simulink model "vector_quantizer_example"  (Simulink 6.0)
settings: Solver=FixedStepDiscrete  SolverMode=SingleTasking  StartTime=0.0  StopTime=0.49  RelTol=1e-3
PreLoadFcn:
  | load mtlb;
undefined symbols (not defined in the file or in its folder): Mag, magnitude, mtlb
libraries: simulink x6, dspquant2 x6, dspsnks4 x5, dspsrcs4 x4, dsparch4 x4, dsplp x4, dspmathops x3, dspmtrx3 x3, dspstat3 x2, dspindex x2, dspsigops x2, dspxfrm3 x1
settings Model: RequirementInfo=9  CovMetricSettings=d  Creator=dshpak  LastModifiedBy=cclarke  ExtModeTrigMode=oneshot  ExtModeArmWhenConnect=off  ExtModeAutoUpdateStatusClock=off  SaveTime=off  SaveOutput=off  SaveFormat=Structure  LimitDataPoints=off  IntegerOverflowMsg=none  BlockReductionOpt=off  ZeroCrossControl=UseLocalSettings  ProdHWDeviceType=Microprocessor  TargetHWChar=2  TargetHWWordLengths=8,16,32,32  RTWMathFcnLibMatFile=iso_c_tmw.mat  RTWOptions="-aEnforceIntegerDowncast=1 -aFoldNonRolledExpr=1 -aInlineInvariantSignals=0 -aInlineParameters=0 -aLocalBlockOutputs=1 -aRollThreshold=5 -aGenerateReport=0 -aGenCodeOnly=0 -aRTWVerbose=1 -aForceParamTrailComments=0 -aGenerateComments=1 -aIgnoreCustomStorageClasses=1 -aIncHierarchyInIds=0 -aMaxRTWIdLen=31 -aShowEliminatedStatements=1 -aPrefixModelToSubsysFcnNames=1 -aIncDataTypeInIds=0 -aInlinedPrmAccess=\"Literals\" -aTargetFcnLib=\"iso_c_tmw.mat\" -aGenerateFullHeader=1 -aIsPILTarget=0 -aExtMode=0 -aExtModeStaticAlloc=0 -aExtModeTesting=0 -aExtModeStaticAllocSize=1000000 -aExtModeTransport=0 -aLogVarNameModifier=\"rt_\" -aRTWCAPISignals=0 -aRTWCAPIParams=0"
settings DataIOCC: LimitDataPoints=off  SaveFormat=Structure  SaveOutput=off  SaveTime=off  SignalLoggingName=sigsOut
settings OptimizationCC: BlockReduction=off  BooleanDataType=off  InlineInvariantSignals=off  MultiInstanced=off
settings FormatCC: IgnoreBidirectionalLines=off
settings DebuggingCC: IntegerOverflowMsg=none
settings HardwareCC: ProdHWDeviceType=Microprocessor  ShiftRightIntArith=on  TargetHWCharacteristics=InheritFromRTWHook
settings CodeAppCC: FileBanners=off
settings GRTTargetCC: TargetFcnLib=iso_c_tmw.mat  IsERTTarget=off

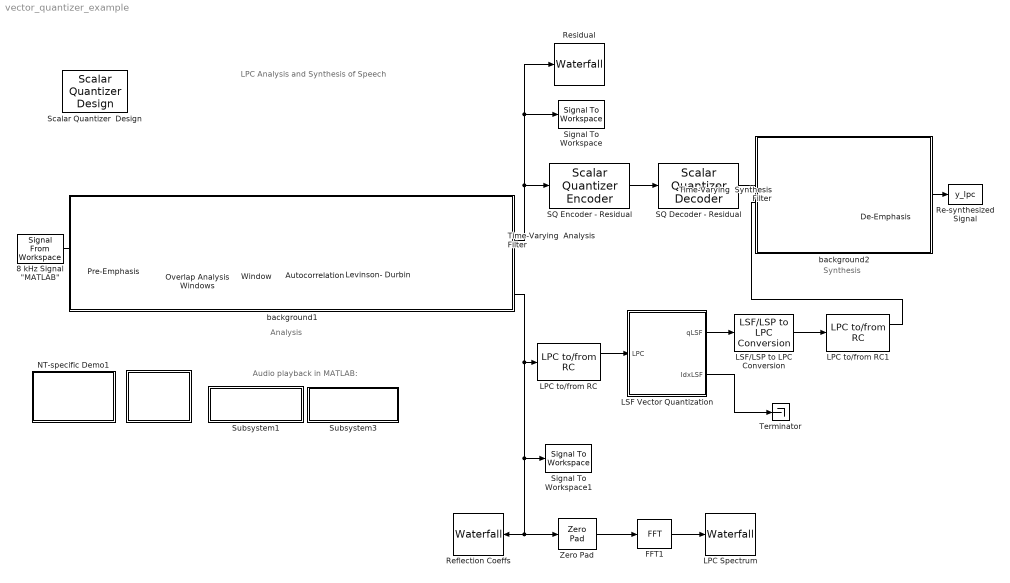
== system vector_quantizer_example ==
  note: LPC Analysis and Synthesis of Speech
  note: Analysis
  note: Synthesis
  note: Audio playback in MATLAB:
  " " : Subsystem
      mask Type: Frame-Based Simulation Info
      mask Display: disp('Info')
  "8 kHz Signal \"MATLAB\"" : dspsrcs4/Signal From Workspace  X=mtlb*0.32  Ts=1/8000  nsamps=80  OutputAfterFinalValue=Setting to zero
  Autocorrelation : dspstat3/Autocorrelation  AllPositiveLags=off  maxlag=12  bias=Biased  domain=Time  roundingMode=Floor  overflowMode=off
  De-Emphasis : dsparch4/Digital Filter  TypePopup=IIR (all poles)  IIRFiltStruct=Direct form II transposed  AllPoleFiltStruct=Direct form  FIRFiltStruct=Direct form  CoeffSource=Specify via dialog  NumCoeffs=[1 -.95]  DenCoeffs=[1 -.95]  BiQuadCoeffs=[1 0.3 0.4 1 0.1 0.2]  LatticeCoeffs=[0.2 0.4]  denIgnore=on  FiltPerSampPopup=One filter per frame  IC=0  ICnum=0  ICden=0  roundingMode=Floor  overflowMode=off
  FFT1 : dspxfrm3/FFT  CompMethod=Table lookup  TableOpt=Speed  BitRevOrder=off  SkipNorm=off  roundingMode=Floor  overflowMode=off
  LPC Spectrum : dspsnks4/Waterfall  TraceProperties=off  NumTraces=10  CMapStr=autumn  TNewest=0.35  TOldest=0.1  HistoryLength=100  HistoryFull=Overwrite  UpdateInterval=1  ExportMode=All visible  MLExportName=ExportData  AutoExport=off  DisplayProperties=off  MouseMode=Orbit  AxisGrid=off  Snapshot=off  Suspend=off  SyncSnapshots=off  OpenScopeAtSimStart=off  FigPos=[452 44 407 353]  CameraView=[89945.9047576273 49093.2447020758 -7462.52930692949 -16.6995606364064 71 5.5 2.5389885178677 -5.30668596526891 0.808418434368868 0.0592442608385446 5.583225828012 14.2 1]  InportDimsHint=[129 1]  AxisProperties=off  AxisColor=[1 1 1]*.9  XLabel=Frequency  YLabel=Mag^2  ZLabel=History  TriggerProperties=off  TrigStartMode=Immediately  TrigStartT=10  TrigStartN=1000  TrigStartFcn=trigPower  TrigStopMode=Never  TrigStopT=0.1  TrigStopN=10  TrigStopFcn=trigend  TrigRearmMode=User-defined  TrigRearmT=0  TrigRearmN=100  TrigRearmFcn=trigrearm  XformProperties=off  XformMode=FFT->Mag dB Fs/2  XformFcn=fliplr  XformExpr=20*log10(abs(u(129:2:end)))
      settings: YMin=-44.6156897764664  YMax=11.2165685036536
  LPC to/from RC : dsplp/LPC to//from RC  conversion=RC to LPC  perr=on  stability=off  error=Replace it with 1
  LPC to/from RC1 : dsplp/LPC to//from RC  conversion=RC to LPC  perr=on  stability=off  error=Replace it with 1
  LSF Vector Quantization : Subsystem
  LSF/LSP to LPC Conversion : dsplp/LSF//LSP to LPC Conversion  input=LSP in range (-1 1)
  Levinson- Durbin : dspsolvers/Levinson-Durbin  coeffOutFcn=K  outP=off  zeroInpHandling=on
  NT-specific Demo1 : Subsystem
      settings: OpenFcn=dsplpc_win32
      mask Type: NT-only Demo
      mask Display: disp('PC/Windows\nLPC Demo')
  Overlap Analysis Windows : dspbuff3/Buffer  N=160  V=80  ic=0
  Pre-Emphasis : dsparch4/Digital Filter  TypePopup=FIR (all zeros)  IIRFiltStruct=Direct form II transposed  AllPoleFiltStruct=Direct form  FIRFiltStruct=Direct form  CoeffSource=Specify via dialog  NumCoeffs=[1 -.95]  DenCoeffs=[1 0.1]  BiQuadCoeffs=[1 0.3 0.4 1 0.1 0.2]  LatticeCoeffs=[0.2 0.4]  denIgnore=on  FiltPerSampPopup=One filter per frame  IC=0  ICnum=0  ICden=0  roundingMode=Floor  overflowMode=off
  Re-synthesized Signal : ToWorkspace  VariableName=y_lpc  SampleTime=-1  SaveFormat=Array
  Reflection Coeffs : dspsnks4/Waterfall  Orientation=left  TraceProperties=off  NumTraces=10  CMapStr=autumn  TNewest=0.7  TOldest=0.1  HistoryLength=50  HistoryFull=Overwrite  UpdateInterval=1  ExportMode=All visible  MLExportName=ExportData2  AutoExport=off  DisplayProperties=off  MouseMode=Orbit  AxisGrid=on  Snapshot=off  Suspend=off  SyncSnapshots=off  OpenScopeAtSimStart=off  FigPos=[35 41 410 358]  CameraView=[73343.0440471642 150383.489958622 -231607.055769344 -0.0735265549347769 7.5 5.5 0.547487828138618 -2.62241953831449 4.03911084299836 0.00240035045613671 1 7.88928028685195 5.25952019123463]  InportDimsHint=[12 1]  AxisProperties=off  AxisColor=[1 1 1]*.9  XLabel=Coefficient  YLabel=RC Amplitude  ZLabel=History  TriggerProperties=off  TrigStartMode=Immediately  TrigStartT=10  TrigStartN=1000  TrigStartFcn=trigPower  TrigStopMode=Never  TrigStopT=0.1  TrigStopN=10  TrigStopFcn=trigend  TrigRearmMode=User-defined  TrigRearmT=0  TrigRearmN=100  TrigRearmFcn=trigrearm  XformProperties=off  XformMode=None  XformFcn=fliplr  XformExpr=20*log10(abs(u(129:2:end)))
      settings: YMin=-1.02418361455266  YMax=0.877130504683106
  Residual : dspsnks4/Waterfall  TraceProperties=off  NumTraces=10  CMapStr=autumn  TNewest=0.7  TOldest=0.1  HistoryLength=50  HistoryFull=Overwrite  UpdateInterval=1  ExportMode=All visible  MLExportName=ExportData2  AutoExport=off  DisplayProperties=off  MouseMode=Orbit  AxisGrid=on  Snapshot=off  Suspend=off  SyncSnapshots=off  OpenScopeAtSimStart=off  FigPos=[524 276 410 358]  CameraView=[62164.2347969079 1792549.89917746 -405278.370332737 -0.097024155318337 44.5 5.5 0.575539043328793 -33.5051317778483 7.57548038023531 0.00104183380472551 1 92.0645761641202 10.3443344004629]  InportDimsHint=[80 1]  AxisProperties=off  AxisColor=[1 1 1]*.9  XLabel=Coefficient  YLabel=Amplitude  ZLabel=History  TriggerProperties=off  TrigStartMode=Immediately  TrigStartT=10  TrigStartN=1000  TrigStartFcn=trigPower  TrigStopMode=Never  TrigStopT=0.1  TrigStopN=10  TrigStopFcn=trigend  TrigRearmMode=User-defined  TrigRearmT=0  TrigRearmN=100  TrigRearmFcn=trigrearm  XformProperties=off  XformMode=None  XformFcn=fliplr  XformExpr=20*log10(abs(u(129:2:end)))
      settings: YMin=-0.580380532484202  YMax=0.386332221847528
  SQ Decoder - Residual : dspquant2/Scalar Quantizer Decoder  Tag=SQDESIGN_GUI_REALIZE_MODEL  CBsource=Specify via dialog  codebook="[-0.52762    -0.50434    -0.48686    -0.48023    -0.47847      -0.471    -0.46439    -0.45511     -0.4483    -0.44149    -0.41351    -0.40777    -0.38649    -0.38257    -0.34459    -0.33656      -0.332    -0.31506     -0.3058    -0.29467    -0.28964    -0.27695    -0.26405    -0.25569    -0.24792    -0.24257    -0.23586    -0.22862     -0.2106    -0.20577    -0.20412    -0.18901    -0.18326    -0.17976    -0.17701    -0.17353    -0.16764    -0.16375    -0.15999    -0.15604    -0.15179    -0.14868    -0.14379    -0.13796    -0.13635    -0.13256    -0.13017    -0.12998    -0.12647    -0.12418    -0.11813     -0.1136    -0.11155    -0.11052    -0.10963    -0.10743    -0.10473    -0.10243     -0.1011   -0.099393   -0.096895   -0.094117   -0.089935   -0.085798   -0.081628   -0.076302   -0.068999   -0.061675   -0.053416   -0.045539   -0.039235   -0.031285   -0.023645   -0.016735   -0.011309  -0.0064137  -0.0017528   0.0031653   0.0083379    0.013857    0.020398      0.0273    0.035732    0.044282    0.051892    0.058205    0.064287    0.068767    0.072477     0.07818    0.082855    0.086893    0.093341     0.10139     0.10818     0.11338     0.12005      0.1266      0.1299     0.13376     0.13746     0.14153     0.14549     0.14866     0.14958     0.15164     0.15552     0.15703     0.15896     0.16211      0.1658     0.16848     0.17145     0.17815      0.1849      0.1891     0.19733     0.20475     0.20935     0.21575     0.22642     0.23266     0.23916     0.24329     0.25005      0.2589     0.27394     0.35121]"  invalidin=Clip  cwdtype=double  outputMode=User-defined  outputWordLength=16  outputFracLength=15
      settings: allowOverrides=off
  SQ Encoder - Residual : dspquant2/Scalar Quantizer Encoder  Tag=SQDESIGN_GUI_REALIZE_MODEL  paramSrc=Specify via dialog  partType=Bounded  BBoundary="[-inf -0.51598     -0.4956    -0.48355    -0.47935    -0.47473    -0.46769    -0.45975     -0.4517     -0.4449     -0.4275    -0.41064    -0.39713    -0.38453    -0.36358    -0.34057    -0.33428    -0.32353    -0.31043    -0.30024    -0.29216    -0.28329     -0.2705    -0.25987     -0.2518    -0.24524    -0.23922    -0.23224    -0.21961    -0.20819    -0.20495    -0.19656    -0.18613    -0.18151    -0.17839    -0.17527    -0.17058    -0.16569    -0.16187    -0.15802    -0.15392    -0.15024    -0.14624    -0.14088    -0.13716    -0.13446    -0.13136    -0.13007    -0.12823    -0.12533    -0.12115    -0.11587    -0.11258    -0.11103    -0.11007    -0.10853    -0.10608    -0.10358    -0.10176    -0.10024   -0.098144   -0.095506   -0.092026   -0.087867   -0.083713   -0.078965   -0.072651   -0.065337   -0.057545   -0.049477   -0.042387    -0.03526   -0.027465    -0.02019   -0.014022  -0.0088614  -0.0040832  0.00070626   0.0057516    0.011097    0.017127    0.023849    0.031516    0.040007    0.048087    0.055049    0.061246    0.066527    0.070622    0.075328    0.080518    0.084874    0.090117    0.097368     0.10479     0.11078     0.11671     0.12332     0.12825     0.13183     0.13561      0.1395     0.14351     0.14707     0.14912     0.15061     0.15358     0.15628       0.158     0.16054     0.16396     0.16714     0.16996      0.1748     0.18152       0.187     0.19321     0.20104     0.20705     0.21255     0.22109     0.22954     0.23591     0.24122     0.24667     0.25447     0.26642     0.31258  +inf]"  UBoundary="[ -0.51598     -0.4956    -0.48355    -0.47935    -0.47473    -0.46769    -0.45975     -0.4517     -0.4449     -0.4275    -0.41064    -0.39713    -0.38453    -0.36358    -0.34057    -0.33428    -0.32353    -0.31043    -0.30024    -0.29216    -0.28329     -0.2705    -0.25987     -0.2518    -0.24524    -0.23922    -0.23224    -0.21961    -0.20819    -0.20495    -0.19656    -0.18613    -0.18151    -0.17839    -0.17527    -0.17058    -0.16569    -0.16187    -0.15802    -0.15392    -0.15024    -0.14624    -0.14088    -0.13716    -0.13446    -0.13136    -0.13007    -0.12823    -0.12533    -0.12115    -0.11587    -0.11258    -0.11103    -0.11007    -0.10853    -0.10608    -0.10358    -0.10176    -0.10024   -0.098144   -0.095506   -0.092026   -0.087867   -0.083713   -0.078965   -0.072651   -0.065337   -0.057545   -0.049477   -0.042387    -0.03526   -0.027465    -0.02019   -0.014022  -0.0088614  -0.0040832  0.00070626   0.0057516    0.011097    0.017127    0.023849    0.031516    0.040007    0.048087    0.055049    0.061246    0.066527    0.070622    0.075328    0.080518    0.084874    0.090117    0.097368     0.10479     0.11078     0.11671     0.12332     0.12825     0.13183     0.13561      0.1395     0.14351     0.14707     0.14912     0.15061     0.15358     0.15628       0.158     0.16054     0.16396     0.16714     0.16996      0.1748     0.18152       0.187     0.19321     0.20104     0.20705     0.21255     0.22109     0.22954     0.23591     0.24122     0.24667     0.25447     0.26642     0.31258  ]"  SearchMethod=Binary  tieBreakRule=Choose the lower index  outQU=off  outQError=off  codebook="[-0.52762    -0.50434    -0.48686    -0.48023    -0.47847      -0.471    -0.46439    -0.45511     -0.4483    -0.44149    -0.41351    -0.40777    -0.38649    -0.38257    -0.34459    -0.33656      -0.332    -0.31506     -0.3058    -0.29467    -0.28964    -0.27695    -0.26405    -0.25569    -0.24792    -0.24257    -0.23586    -0.22862     -0.2106    -0.20577    -0.20412    -0.18901    -0.18326    -0.17976    -0.17701    -0.17353    -0.16764    -0.16375    -0.15999    -0.15604    -0.15179    -0.14868    -0.14379    -0.13796    -0.13635    -0.13256    -0.13017    -0.12998    -0.12647    -0.12418    -0.11813     -0.1136    -0.11155    -0.11052    -0.10963    -0.10743    -0.10473    -0.10243     -0.1011   -0.099393   -0.096895   -0.094117   -0.089935   -0.085798   -0.081628   -0.076302   -0.068999   -0.061675   -0.053416   -0.045539   -0.039235   -0.031285   -0.023645   -0.016735   -0.011309  -0.0064137  -0.0017528   0.0031653   0.0083379    0.013857    0.020398      0.0273    0.035732    0.044282    0.051892    0.058205    0.064287    0.068767    0.072477     0.07818    0.082855    0.086893    0.093341     0.10139     0.10818     0.11338     0.12005      0.1266      0.1299     0.13376     0.13746     0.14153     0.14549     0.14866     0.14958     0.15164     0.15552     0.15703     0.15896     0.16211      0.1658     0.16848     0.17145     0.17815      0.1849      0.1891     0.19733     0.20475     0.20935     0.21575     0.22642     0.23266     0.23916     0.24329     0.25005      0.2589     0.27394     0.35121]"  outStatus=off  invalidin=Clip  idtype=int32  roundingMode=Nearest  overflowMode=on
  Scalar Quantizer  Design : dspquant2/Scalar Quantizer  Design
  Signal To Workspace : dspsnks4/Signal To Workspace  VariableName=E  FrameMode=Concatenate frames (2-D array)
  Signal To Workspace1 : dspsnks4/Signal To Workspace  VariableName=K  FrameMode=Concatenate frames (2-D array)
  Subsystem1 : Subsystem
      settings: OpenFcn=if exist('mtlb','var'), sound(mtlb*0.32,8000); else errordlg('Data not found in workspace - reload demo model.','DSP Blockset Demo Error'); end
      mask Display: disp('Original\nSignal')
  Subsystem3 : Subsystem
      settings: OpenFcn=if exist('y_lpc','var'), sound(y_lpc,8000); else errordlg('You must run the simulation first.','DSP Blockset Demo Error'); end
      mask Display: disp('Processed\nSignal')
  Terminator : Terminator
  Time-Varying  Analysis Filter : dsparch4/Digital Filter  TypePopup=FIR (all zeros)  IIRFiltStruct=Direct form II transposed  AllPoleFiltStruct=Direct form  FIRFiltStruct=Lattice MA  CoeffSource=Input port(s)  NumCoeffs=[1 -.95]  DenCoeffs=[1 0.1]  BiQuadCoeffs=[1 0.3 0.4 1 0.1 0.2]  LatticeCoeffs=[0.2 0.4]  denIgnore=on  FiltPerSampPopup=One filter per frame  IC=0  ICnum=0  ICden=0  roundingMode=Floor  overflowMode=off
  Time-Varying  Synthesis Filter : dsparch4/Digital Filter  TypePopup=IIR (all poles)  IIRFiltStruct=Direct form II transposed  AllPoleFiltStruct=Lattice AR  FIRFiltStruct=Direct form  CoeffSource=Input port(s)  NumCoeffs=[1 -.95]  DenCoeffs=[1 0.1]  BiQuadCoeffs=[1 0.3 0.4 1 0.1 0.2]  LatticeCoeffs=[0.2 0.4]  denIgnore=on  FiltPerSampPopup=One filter per frame  IC=0  ICnum=0  ICden=0  roundingMode=Floor  overflowMode=off
  Window : dspsigops/Window Function  winmode=Apply window to input  wintype=Hamming  sampmode=Continuous  samptime=1  N=64  Rs=50  beta=10  winsamp=Symmetric  UserWindow=hamming  OptParams=off  UserParams={1.0}  dataType=double  wordLen=16  udDataType=sfix(16)  fracBitsMode=Best precision  numFracBits=15  roundingMode=Floor  overflowMode=off
  Zero Pad : dspsigops/Zero Pad  padSigAt=End  zpadAlong=Columns  padNumOutRowsSpecMethod=User-specified  numOutRows=256  padNumOutColsSpecMethod=User-specified  numOutCols=1  trunc_flag=None
  background1 : Subsystem
      mask Display: disp('')
  background2 : Subsystem
      mask Display: disp('')
  wires:
  "8 kHz Signal \"MATLAB\""/1 -> Pre-Emphasis/1
  Pre-Emphasis/1 -> Overlap Analysis Windows/1, Time-Varying  Analysis Filter/1
  Overlap Analysis Windows/1 -> Window/1
  Autocorrelation/1 -> Levinson- Durbin/1
  Window/1 -> Autocorrelation/1
  Time-Varying  Analysis Filter/1 -> Residual/1, Signal To Workspace/1, SQ Encoder - Residual/1
  Levinson- Durbin/1 -> Time-Varying  Analysis Filter/2, Reflection Coeffs/1, Zero Pad/1, Signal To Workspace1/1, LPC to/from RC/1
  Time-Varying  Synthesis Filter/1 -> De-Emphasis/1
  De-Emphasis/1 -> Re-synthesized Signal/1
  Zero Pad/1 -> FFT1/1
  FFT1/1 -> LPC Spectrum/1
  SQ Encoder - Residual/1 -> SQ Decoder - Residual/1
  SQ Decoder - Residual/1 -> Time-Varying  Synthesis Filter/1
  LSF Vector Quantization/2(IdxLSF) -> Terminator/1
  LPC to/from RC/1 -> LSF Vector Quantization/1(LPC)
  LSF Vector Quantization/1(qLSF) -> LSF/LSP to LPC Conversion/1
  LSF/LSP to LPC Conversion/1 -> LPC to/from RC1/1
  LPC to/from RC1/1 -> Time-Varying  Synthesis Filter/2

== system vector_quantizer_example/  ==
  note: LPC Analysis and Synthesis of Speech
      |
      | This demo consists of two parts,  analysis and synthesis. The analysis part
      | is found in the transmitter section of a system. Using the original speech signal, parameters
      | (reflection coefficients) and the residual signal are extracted from it, and then transmitted over
      | a channel. The synthesis part , which is found in the receiver section of the system, reconstructs
      | the original signal using those parameters and the residual signal.
      |
      | In this simulation , the speech signal is divided into
      | frames of size 20 ms (160 samples) , with an overlap of 10 ms (80 samples).Each frame
      | is then windowed using a hamming window, 11th order autocorrelation coefficients
      | are found and then the reflection coefficients (11th order) are calculated from the autocorrelation
      | coefficients, using the Levinson-Durbin algorithm. The original speech signal is passed through an
      |  analysis-filter which is basically an all-zero filter with coefficients as the reflection coefficients
      | obtained above. The output of the filter is the residual signal. This residual signal is then
      | passed through a synthesis-filter which is basically an all-pole filter, again with coefficients as the
      | reflection coefficients (Synthesis filter is just the inverse of Analysis filter). The output of the
      | synthesis filter is the original signal.

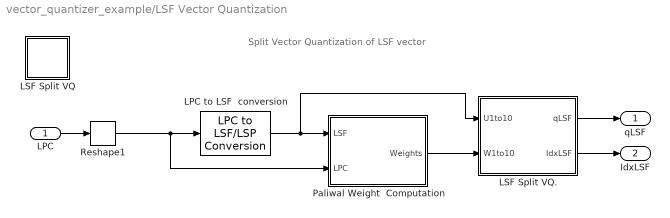
== system vector_quantizer_example/LSF Vector Quantization ==
  note: Split Vector Quantization of LSF vector
  LPC : Inport
  LPC to LSF  conversion : dsplp/LPC to LSF//LSP Conversion  output=LSF in range (0 pi)  NSteps=64  NBisects=4  RootStatus=off  correction=off  lastLSP=off  error=Ignore
  LSF Split VQ : Subsystem  mask(DocBlock){ECoderFlag=, DocumentType=Text}
      mask prompts: ECoderFlag "RTW Embedded Coder Flag"; DocumentType "Document Type"
      mask help: Use this block to save long descriptive text with the model. Double-clicking the block will open an editor.
      settings: CopyFcn=docblock('breaklink',gcb);  DeleteFcn=docblock('close_document',gcb);  PreSaveFcn=docblock('save_document',gcb);  OpenFcn=docblock('edit_document',gcb);
      mask StyleString: edit,popup(Text|RTF|HTML)
      mask Display:
      | plot([.8 0 0 1 1 .8 .8 1],[1 1 0 0 .8 1 .8 .8]);
      | text(.5,.5,'DOC','horizontalalignment','center');
  LSF Split VQ. : Subsystem
  Paliwal Weight  Computation : Subsystem
  Reshape1 : simulink/Math Operations/Reshape  OutputDimensionality=Column vector  OutputDimensions=[1,1]
  qLSF : Outport
  IdxLSF : Outport  Port=2
  wires:
  LPC/1 -> Reshape1/1
  Paliwal Weight  Computation/1(Weights) -> LSF Split VQ./2(W1to10)
  Reshape1/1 -> LPC to LSF  conversion/1, Paliwal Weight  Computation/2(LPC)
  LPC to LSF  conversion/1 -> Paliwal Weight  Computation/1(LSF), LSF Split VQ./1(U1to10)
  LSF Split VQ./1(qLSF) -> qLSF/1
  LSF Split VQ./2(IdxLSF) -> IdxLSF/1

== system vector_quantizer_example/NT-specific Demo1 ==

== system vector_quantizer_example/Subsystem1 ==

== system vector_quantizer_example/Subsystem3 ==

== system vector_quantizer_example/background1 ==

== system vector_quantizer_example/background2 ==

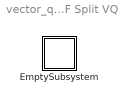
== system vector_quantizer_example/LSF Vector Quantization/LSF Split VQ ==
  EmptySubsystem : Subsystem

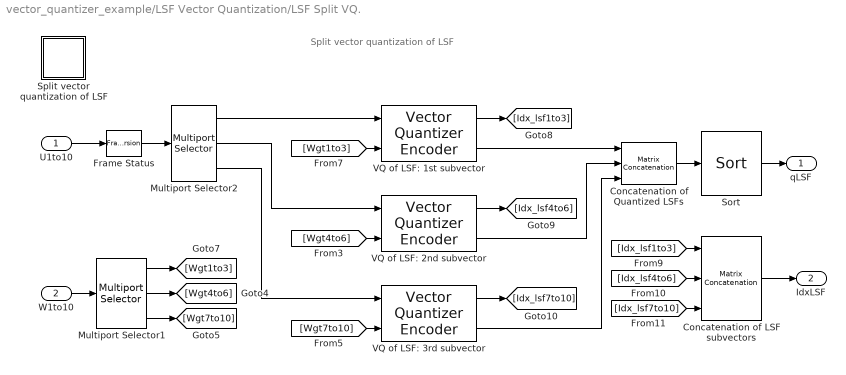
== system vector_quantizer_example/LSF Vector Quantization/LSF Split VQ. ==
  note: Split vector quantization of LSF
  U1to10 : Inport
  W1to10 : Inport  Port=2
  Concatenation of LSF subvectors : simulink/Math Operations/Matrix Concatenation  numInports=3  catMethod=Horizontal
  Concatenation of Quantized LSFs : simulink/Math Operations/Matrix Concatenation  numInports=3  catMethod=Vertical
  Frame Status : FrameConversion
  Multiport Selector1 : dspindex/Multiport Selector  rowsOrCols=Rows  idxCellArray={1:3,4:6,7:10}  idxErrMode=Clip Index
  Multiport Selector2 : dspindex/Multiport Selector  rowsOrCols=Rows  idxCellArray={1:3,4:6,7:10}  idxErrMode=Clip Index
  Sort : dspstat3/Sort  otype=Value  dir=Ascending  sortAlg=Quick sort  roundingMode=Floor  overflowMode=off
  Split vector quantization of LSF : Subsystem  mask(DocBlock){ECoderFlag=, DocumentType=Text}
      mask prompts: ECoderFlag "RTW Embedded Coder Flag"; DocumentType "Document Type"
      mask help: Use this block to save long descriptive text with the model. Double-clicking the block will open an editor.
      settings: CopyFcn=docblock('breaklink',gcb);  DeleteFcn=docblock('close_document',gcb);  PreSaveFcn=docblock('save_document',gcb);  OpenFcn=docblock('edit_document',gcb);
      mask StyleString: edit,popup(Text|RTF|HTML)
      mask Display:
      | plot([.8 0 0 1 1 .8 .8 1],[1 1 0 0 .8 1 .8 .8]);
      | text(.5,.5,'DOC','horizontalalignment','center');
  VQ of LSF: 1st subvector : dspquant2/Vector Quantizer Encoder  CBsource=Specify via dialog  codebook=CB_lsf1to3_10bit  distMeasure=Weighted squared error  wgtSrc=Input port  weights=[1 1 1]  tieBreakRule=Choose the lower index  outQU=on  outQError=off  idtype=int32  roundingMode=Floor  overflowMode=off
      settings: allowOverrides=off
  VQ of LSF: 2nd subvector : dspquant2/Vector Quantizer Encoder  CBsource=Specify via dialog  codebook=CB_lsf4to6_10bit  distMeasure=Weighted squared error  wgtSrc=Input port  weights=[1 1 1]  tieBreakRule=Choose the lower index  outQU=on  outQError=off  idtype=int32  roundingMode=Floor  overflowMode=off
      settings: allowOverrides=off
  VQ of LSF: 3rd subvector : dspquant2/Vector Quantizer Encoder  CBsource=Specify via dialog  codebook=CB_lsf7to10_10bit  distMeasure=Weighted squared error  wgtSrc=Input port  weights=[1 1 1]  tieBreakRule=Choose the lower index  outQU=on  outQError=off  idtype=int32  roundingMode=Floor  overflowMode=off
      settings: allowOverrides=off
  qLSF : Outport
  IdxLSF : Outport  Port=2
  wires:
  VQ of LSF: 1st subvector/2 -> Concatenation of Quantized LSFs/1
  VQ of LSF: 1st subvector/1 -> [Idx_lsf1to3]
  Multiport Selector2/2 -> VQ of LSF: 2nd subvector/1
  Multiport Selector2/3 -> VQ of LSF: 3rd subvector/1
  Multiport Selector1/2 -> [Wgt4to6]
  Multiport Selector1/3 -> [Wgt7to10]
  VQ of LSF: 2nd subvector/1 -> [Idx_lsf4to6]
  [Wgt7to10] -> VQ of LSF: 3rd subvector/2
  VQ of LSF: 3rd subvector/1 -> [Idx_lsf7to10]
  VQ of LSF: 2nd subvector/2 -> Concatenation of Quantized LSFs/2
  Concatenation of Quantized LSFs/1 -> Sort/1
  VQ of LSF: 3rd subvector/2 -> Concatenation of Quantized LSFs/3
  [Wgt4to6] -> VQ of LSF: 2nd subvector/2
  Multiport Selector1/1 -> [Wgt1to3]
  [Wgt1to3] -> VQ of LSF: 1st subvector/2
  [Idx_lsf1to3] -> Concatenation of LSF subvectors/1
  [Idx_lsf4to6] -> Concatenation of LSF subvectors/2
  [Idx_lsf7to10] -> Concatenation of LSF subvectors/3
  W1to10/1 -> Multiport Selector1/1
  U1to10/1 -> Frame Status/1
  Sort/1 -> qLSF/1
  Concatenation of LSF subvectors/1 -> IdxLSF/1
  Frame Status/1 -> Multiport Selector2/1
  Multiport Selector2/1 -> VQ of LSF: 1st subvector/1

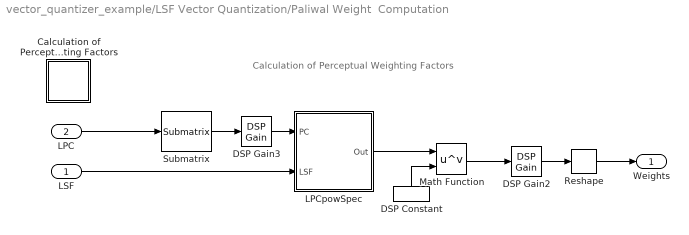
== system vector_quantizer_example/LSF Vector Quantization/Paliwal Weight  Computation ==
  note: Calculation of Perceptual Weighting Factors
  LSF : Inport
  LPC : Inport  Port=2
  Calculation of Perceptual  Weighting Factors : Subsystem  mask(DocBlock){ECoderFlag=, DocumentType=Text}
      mask prompts: ECoderFlag "RTW Embedded Coder Flag"; DocumentType "Document Type"
      mask help: Use this block to save long descriptive text with the model. Double-clicking the block will open an editor.
      settings: CopyFcn=docblock('breaklink',gcb);  DeleteFcn=docblock('close_document',gcb);  PreSaveFcn=docblock('save_document',gcb);  OpenFcn=docblock('edit_document',gcb);
      mask StyleString: edit,popup(Text|RTF|HTML)
      mask Display:
      | plot([.8 0 0 1 1 .8 .8 1],[1 1 0 0 .8 1 .8 .8]);
      | text(.5,.5,'DOC','horizontalalignment','center');
  DSP Constant : dspsrcs4/DSP Constant  Orientation=up  Value=0.15  SampleMode=Discrete  discreteOutput=Sample-based  continuousOutput=Sample-based  sampTime=-1  framePeriod=-1  dataType=Inherit from 'Constant value'  wordLen=16  udDataType=sfix(16)  fracBitsMode=Best precision  numFracBits=15  InterpretAs1D=off  Ts=-1  FramebasedOutput=off
      settings: AttributesFormatString=\n\n\n\n
  DSP Gain2 : dspmathops/DSP Gain  gainValue=[ones(1,8) 0.8 0.4]  roundingMode=Floor  overflowMode=off
  DSP Gain3 : dspmathops/DSP Gain  gainValue=-1  roundingMode=Floor  overflowMode=off
  LPCpowSpec : Subsystem
  Math Function : Math  Operator=pow
  Reshape : simulink/Math Operations/Reshape  OutputDimensionality=Column vector  OutputDimensions=[1,1]
  Submatrix : dspmtrx3/Submatrix  RowSpan=Range of rows  RowStartMode=Index  RowStartIndex=2  RowEndMode=Last  RowEndIndex=1  ColSpan=All columns  ColStartMode=First  ColStartIndex=1  ColEndMode=Last  ColEndIndex=1
  Weights : Outport
  wires:
  LPCpowSpec/1(Out) -> Math Function/1
  DSP Constant/1 -> Math Function/2
  Math Function/1 -> DSP Gain2/1
  DSP Gain2/1 -> Reshape/1
  LSF/1 -> LPCpowSpec/2(LSF)
  Reshape/1 -> Weights/1
  Submatrix/1 -> DSP Gain3/1
  LPC/1 -> Submatrix/1
  DSP Gain3/1 -> LPCpowSpec/1(PC)

== system vector_quantizer_example/LSF Vector Quantization/LSF Split VQ/EmptySubsystem ==

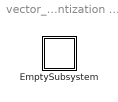
== system vector_quantizer_example/LSF Vector Quantization/LSF Split VQ./Split vector quantization of LSF ==
  EmptySubsystem : Subsystem

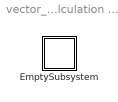
== system vector_quantizer_example/LSF Vector Quantization/Paliwal Weight  Computation/Calculation of Perceptual  Weighting Factors ==
  EmptySubsystem : Subsystem

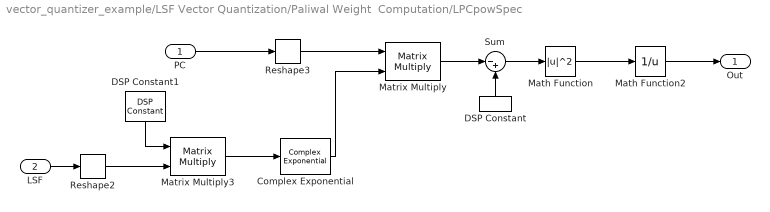
== system vector_quantizer_example/LSF Vector Quantization/Paliwal Weight  Computation/LPCpowSpec ==
  PC : Inport
  LSF : Inport  Port=2
  Complex Exponential : dspmathops/Complex Exponential
  DSP Constant : dspsrcs4/DSP Constant  Orientation=up  Value=1  SampleMode=Discrete  discreteOutput=Frame-based  continuousOutput=Sample-based  sampTime=-1  framePeriod=-1  dataType=Inherit from 'Constant value'  wordLen=16  udDataType=sfix(16)  fracBitsMode=Best precision  numFracBits=15  InterpretAs1D=off  Ts=-1  FramebasedOutput=on
      settings: AttributesFormatString=\n\n\n\n
  DSP Constant1 : dspsrcs4/DSP Constant  Orientation=down  Value=[1:10]'  SampleMode=Discrete  discreteOutput=Frame-based  continuousOutput=Sample-based  sampTime=-1  framePeriod=-1  dataType=Inherit from 'Constant value'  wordLen=16  udDataType=sfix(16)  fracBitsMode=Best precision  numFracBits=15  InterpretAs1D=off  Ts=-1  FramebasedOutput=on
      settings: AttributesFormatString=\n\n\n\n
  Math Function : Math  Operator=magnitude^2
  Math Function2 : Math  Operator=reciprocal
  Matrix Multiply : dspmtrx3/Matrix Multiply  numInputPorts=2  OptimizationLevel=None
  Matrix Multiply3 : dspmtrx3/Matrix Multiply  numInputPorts=2  OptimizationLevel=None
  Reshape2 : simulink/Math Operations/Reshape  OutputDimensionality=Row vector  OutputDimensions=[1,1]
  Reshape3 : simulink/Math Operations/Reshape  OutputDimensionality=Row vector  OutputDimensions=[1,1]
  Sum : Sum  Inputs=|-+  SaturateOnIntegerOverflow=on
  Out : Outport
  wires:
  Math Function2/1 -> Out/1
  Matrix Multiply/1 -> Sum/1
  PC/1 -> Reshape3/1
  Complex Exponential/1 -> Matrix Multiply/2
  Math Function/1 -> Math Function2/1
  Sum/1 -> Math Function/1
  DSP Constant/1 -> Sum/2
  Reshape3/1 -> Matrix Multiply/1
  LSF/1 -> Reshape2/1
  Reshape2/1 -> Matrix Multiply3/2
  DSP Constant1/1 -> Matrix Multiply3/1
  Matrix Multiply3/1 -> Complex Exponential/1

== system vector_quantizer_example/LSF Vector Quantization/LSF Split VQ./Split vector quantization of LSF/EmptySubsystem ==

== system vector_quantizer_example/LSF Vector Quantization/Paliwal Weight  Computation/Calculation of Perceptual  Weighting Factors/EmptySubsystem ==
